simulink model "Counter_UP"  (R2018a)
settings: Solver=VariableStepAuto  StartTime=0.0  StopTime=10.0  RelTol=1e-3
settings Model: Creator=user  LastModifiedBy=user

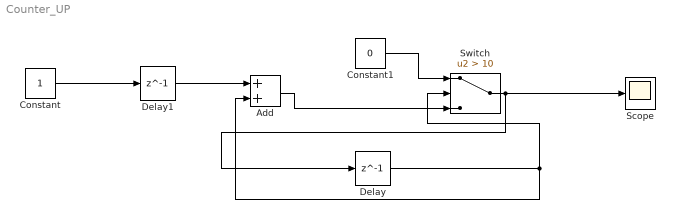
== system Counter_UP ==
  Add : Sum
  Constant : Constant
  Constant1 : Constant  Value=0
  Delay : Delay  DelayLength=1
  Delay1 : Delay  DelayLength=1
  Scope : Scope
  Switch : Switch  Criteria=u2 > Threshold  Threshold=10
  wires:
  Constant/1 -> Delay1/1
  Add/1 -> Switch/3
  Constant1/1 -> Switch/1
  Switch/1 -> Delay/1, Scope/1
  Delay/1 -> Add/2, Switch/2
  Delay1/1 -> Add/1
